simulink model "expt_1"  (R2025a)
settings: Solver=VariableStepAuto  StartTime=0.0  StopTime=1  RelTol=1e-3
values from neighbouring files (symbols this model uses):
  A = 69.7    [RES_EXP_04.m]
libraries: spsSeriesRLCBranchLib x2, spsCurrentMeasurementLib x1, spsPermanentMagnetSynchronousMachineLib x1, spsThreePhaseVIMeasurementLib x1, spsUniversalBridgeLib x1, spsVoltageMeasurementLib x1, spsWindTurbineLib x1, sps_lib x1
settings Model: Creator=kanis  LastModifiedBy=Sheebha

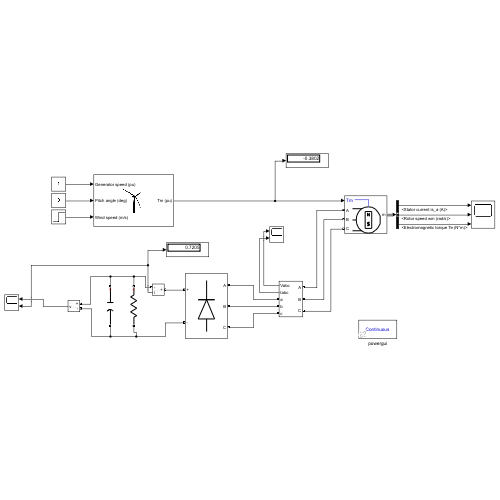
[thumbnail: Simulink's stored preview of the top-level diagram]
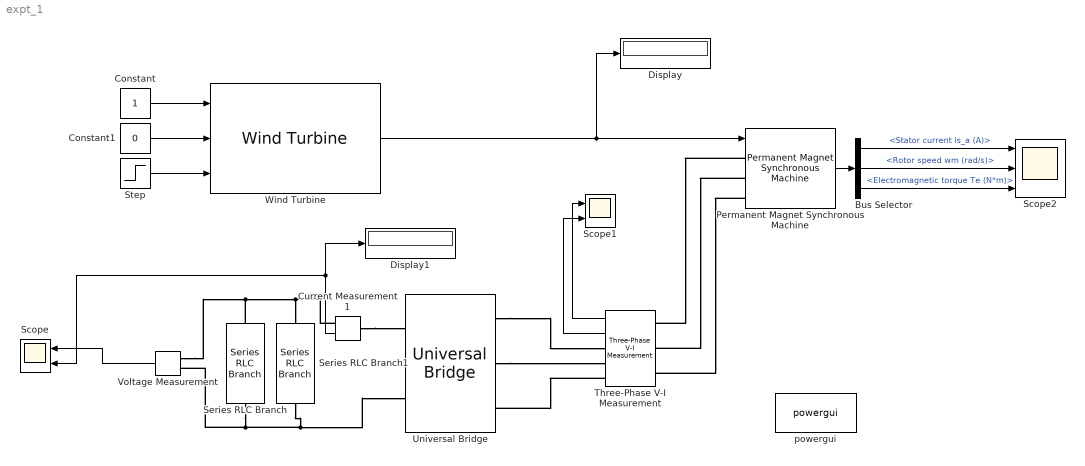
== system expt_1 ==
  Bus Selector : BusSelector  OutputSignals=Stator current is_a (A),Rotor speed wm (rad/s),Electromagnetic torque Te (N*m)
  Constant : Constant
  Constant1 : Constant  Value=0
  Current Measurement1 : spsCurrentMeasurementLib/Current Measurement  PhasorSimulation=off  OutputType=Complex  PSBequivalent=0
  Display : Display
  Display1 : Display
  Permanent Magnet Synchronous Machine : spsPermanentMagnetSynchronousMachineLib/Permanent Magnet Synchronous Machine  NbPhases=3  FluxDistribution=Sinusoidal  RotorType=Round  MechanicalLoad=Torque Tm  PresetModel="01:  0.8 Nm 300 Vdc 3000 RPM - 0.8 Nm"  ShowDetailedParameters=on  MeasurementBus=off  Resistance=18.7  Inductance=8.5e-3  dqInductances=[8.5e-3,8.5e-3]  La=0.02682  MachineConstant=Flux linkage established by magnets (V.s)  Flux=0.1716  VoltageCst=62.2496  TorqueCst=0.5148  Flat=120  Mechanical=[2.26e-05 1.349e-05 2 0]  PolePairs=2  InitialConditions=[0,0, 0,0]  InitialConditions5ph=[0 0 0 0 0 0]  RefAngle=90 degrees behind phase A axis (modified Park)  IterativeDiscreteModel=Trapezoidal non iterative  TsBlock=-1  TsPowergui=0
  Scope : Scope  NumInputPorts=2
      settings: ActiveDisplayYMinimum=-0.091125987718907189  ActiveDisplayYMaximum=0.82013388947016486  YLabel=CURRENT(A)
  Scope1 : Scope  NumInputPorts=2
      settings: ActiveDisplayYMinimum=-818.42622434801046  ActiveDisplayYMaximum=818.42653396486753  YLabel=VOLTAGE(V)
  Scope2 : Scope  NumInputPorts=3
      settings: ActiveDisplayString=3  ActiveDisplayYMinimum=-0.46175493396540529  ActiveDisplayYMaximum=0.051306103773933909  YLabel=TORQUE(Nm)  DataLoggingVariableName=ScopeData2
  Series RLC Branch : spsSeriesRLCBranchLib/Series RLC Branch  LConnTagsString=__new0  RConnTagsString=__new0  BranchType=C  Resistance=1  Inductance=1e-3  SetiL0=off  InitialCurrent=0  Capacitance=50e-6  Setx0=off  InitialVoltage=0  Measurements=None
  Series RLC Branch1 : spsSeriesRLCBranchLib/Series RLC Branch  LConnTagsString=__new0  RConnTagsString=__new0  BranchType=R  Resistance=1000  Inductance=1e-3  SetiL0=off  InitialCurrent=0  Capacitance=1e-6  Setx0=off  InitialVoltage=0  Measurements=None
  Step : Step  Time=0.5  Before=8  After=10  SampleTime=0
  Three-Phase V-I Measurement : spsThreePhaseVIMeasurementLib/Three-Phase V-I Measurement  VoltageMeasurement=phase-to-phase  SetLabelV=off  LabelV=Vabc  Vpu=off  VpuLL=off  CurrentMeasurement=yes  SetLabelI=off  LabelI=Iabc  Ipu=off  Pbase=100e6  Vbase=500e3  OutputType=Complex  PhasorSimulation=off  PSBequivalent=0
  Universal Bridge : spsUniversalBridgeLib/Universal Bridge  Arms=3  SnubberResistance=1e5  SnubberCapacitance=inf  Device=Diodes  Ron=1e-3  Lon=0  ForwardVoltages="[  0  0  ]"  ForwardVoltage=0  GTOparameters=[ 10e-6 , 20e-6 ]  IGBTparameters=[ 1e-6 , 2e-6 ]  Measurements=None  Measurements_2=None  converterType=Rectifier
  Voltage Measurement : spsVoltageMeasurementLib/Voltage Measurement  PhasorSimulation=off  OutputType=Complex  PSBequivalent=0
  Wind Turbine : spsWindTurbineLib/Wind Turbine  Pnom=1.5e6  Pelec_base=1.5e6/0.9  wind_base=12  P_wind_base=0.73  speed_nom=1.2  pitch_angle=0  c1_c6="[0.51763          116          0.4            5           21     0.006795]"  cp_nom=0.48  lambda_nom=8.1
  powergui : sps_lib/powergui  Priority=1  SimulationMode=Continuous  SampleTime=50e-4  frequency=60  Iterations=50  frequencyindice=0  Pbase=100e6  ErrMax=1e-4  UnitsV=kV  UnitsW=MW  buscounter=0  FunctionMessages=off  echomessages=off  EnableUseOfTLC=off  CurrentSourceSwitches=off  DisableSnubberDevices=off  DisableRonSwitches=off  DisableVfSwitches=off  DisplayEquations=off  AutomaticDiscreteSolvers=off  SolverType=Tustin/Backward Euler (TBE)  Interpol=off  ExternalGateDelay=off  methode=off  Ts=100  x0status=blocks  SPID=on  SwTol=0  HookPort=off  NonlinearTolerance=1e-4  nMaxIteration=100  ContinueOnMaxIteration=off  RestoreLinks=warning  ResistiveCurrentMeasurement=off  Frange=[0:2:500]  Ylog=off  Xlog=on  ShowGrid=off  save=off  variable=ZData  structure=0  ZoomFFT=off  StartTime=0.0  cycles=1  DisplayStyle=1  fundamental=60  FreqAxis=off  MaxFrequency=1000  frequencyindicesteady=1  RmsSteady=1  display=off
  wires:
  Step/1 -> Wind Turbine/3
  Constant1/1 -> Wind Turbine/2
  Constant/1 -> Wind Turbine/1
  Wind Turbine/1 -> Permanent Magnet Synchronous Machine/1, Display/1
  Three-Phase V-I Measurement/1 -> Scope1/1
  Three-Phase V-I Measurement/2 -> Scope1/2
  Voltage Measurement/1 -> Scope/1
  Permanent Magnet Synchronous Machine/1 -> Bus Selector/1
  Bus Selector/1 -> Scope2/1  "<Stator current is_a (A)>"
  Bus Selector/2 -> Scope2/2  "<Rotor speed wm (rad/s)>"
  Bus Selector/3 -> Scope2/3  "<Electromagnetic torque Te (N*m)>"
  Current Measurement1/1 -> Display1/1, Scope/2
  connections:
  Permanent Magnet Synchronous Machine/LConn1 -- Three-Phase V-I Measurement/LConn1
  Permanent Magnet Synchronous Machine/LConn2 -- Three-Phase V-I Measurement/LConn2
  Permanent Magnet Synchronous Machine/LConn3 -- Three-Phase V-I Measurement/LConn3
  Universal Bridge/LConn1 -- Three-Phase V-I Measurement/RConn1
  Universal Bridge/LConn2 -- Three-Phase V-I Measurement/RConn2
  Three-Phase V-I Measurement/RConn3 -- Universal Bridge/LConn3
  Voltage Measurement/LConn1 -- Series RLC Branch/LConn1 -- Series RLC Branch1/LConn1 -- Current Measurement1/RConn1
  Series RLC Branch1/RConn1 -- Universal Bridge/RConn2 -- Voltage Measurement/LConn2 -- Series RLC Branch/RConn1
  Current Measurement1/LConn1 -- Universal Bridge/RConn1
